simulink model "tx2"  (R2022a)
settings: Solver=FixedStepDiscrete  StartTime=0.0  StopTime=3.1e6  FixedStep=1  RelTol=1e-3
undefined symbols (not defined in the file or in its folder): rom_bf1, rom_bf2, rom_bf3, rom_bf4, rom_bf5, rom_bf6, rom_bf7, rom_bf8, rom_pilot_tt
libraries: hdlsllib x809, whdlutilities x460, whdlmod x104, whdledac x26, simulink x3
(part 10 of 27)

== system tx2/Subsystem11/bit_level/valid_recover ==
  data_in : Inport
  start_in : Inport  Port=2
  end_in : Inport  Port=3
  Constant : Constant  OutDataTypeStr=boolean
  Constant1 : Constant  Value=0  OutDataTypeStr=boolean
  Constant2 : Constant  OutDataTypeStr=boolean
  Constant3 : Constant  Value=0  OutDataTypeStr=boolean
  Constant4 : Constant  OutDataTypeStr=boolean
  Constant5 : Constant  Value=0  OutDataTypeStr=boolean
  Delay{,1..4} (5 alike) : Delay  DelayLength=1  InitialCondition=0
  Logical Operator1 : Logic  Operator=OR  AllPortsSameDT=off  OutDataTypeStr=boolean
  Logical Operator2 : Logic  AllPortsSameDT=off  OutDataTypeStr=boolean
  Switch : Switch  Criteria=u2 ~= 0  SaturateOnIntegerOverflow=off  InputSameDT=off
  Switch1 : Switch  Criteria=u2 ~= 0  SaturateOnIntegerOverflow=off  InputSameDT=off
  Switch2 : Switch  Criteria=u2 ~= 0  SaturateOnIntegerOverflow=off  InputSameDT=off
  data_out : Outport  VectorParamsAs1DForOutWhenUnconnected=off
  start_out : Outport  Port=2  VectorParamsAs1DForOutWhenUnconnected=off
  end_out : Outport  Port=3  VectorParamsAs1DForOutWhenUnconnected=off
  valid_out : Outport  Port=4  VectorParamsAs1DForOutWhenUnconnected=off
  wires:
  Delay4/1 -> data_out/1
  data_in/1 -> Delay4/1
  Delay1/1 -> Delay2/1, end_out/1
  end_in/1 -> Delay1/1
  Constant1/1 -> Switch/3
  Logical Operator2/1 -> Delay3/1, valid_out/1
  Constant3/1 -> Switch1/1
  start_in/1 -> Delay/1
  Constant4/1 -> Switch2/1
  Constant5/1 -> Switch2/3
  Delay3/1 -> Switch2/2
  Switch2/1 -> Logical Operator1/1
  Logical Operator1/1 -> Logical Operator2/1
  Delay2/1 -> Switch1/2
  Delay/1 -> Switch/2, start_out/1
  Switch1/1 -> Logical Operator2/2
  Switch/1 -> Logical Operator1/2
  Constant2/1 -> Switch1/3
  Constant/1 -> Switch/1

== system tx2/Subsystem12/BF/rom_bf1 ==
  address : Inport
  read_en : Inport  Port=2
  HDL ROM : Subsystem
  InputReg : Delay  DelayLength=1  ShowEnablePort=on
      settings: InputPortMap=u0,e6
  data_out : Outport
  wires:
  address/1 -> InputReg/1
  InputReg/1 -> HDL ROM/1(rom_address)
  read_en/1 -> InputReg/2
  HDL ROM/1(data_out) -> data_out/1

== system tx2/Subsystem12/BF/rom_bf2 ==
  address : Inport
  read_en : Inport  Port=2
  HDL ROM : Subsystem
  InputReg : Delay  DelayLength=1  ShowEnablePort=on
      settings: InputPortMap=u0,e6
  data_out : Outport
  wires:
  HDL ROM/1(data_out) -> data_out/1
  read_en/1 -> InputReg/2
  InputReg/1 -> HDL ROM/1(rom_address)
  address/1 -> InputReg/1

== system tx2/Subsystem12/BF/rom_bf3 ==
  address : Inport
  read_en : Inport  Port=2
  HDL ROM : Subsystem
  InputReg : Delay  DelayLength=1  ShowEnablePort=on
      settings: InputPortMap=u0,e6
  data_out : Outport
  wires:
  address/1 -> InputReg/1
  InputReg/1 -> HDL ROM/1(rom_address)
  read_en/1 -> InputReg/2
  HDL ROM/1(data_out) -> data_out/1

== system tx2/Subsystem12/BF/rom_bf4 ==
  address : Inport
  read_en : Inport  Port=2
  HDL ROM : Subsystem
  InputReg : Delay  DelayLength=1  ShowEnablePort=on
      settings: InputPortMap=u0,e6
  data_out : Outport
  wires:
  HDL ROM/1(data_out) -> data_out/1
  read_en/1 -> InputReg/2
  InputReg/1 -> HDL ROM/1(rom_address)
  address/1 -> InputReg/1

== system tx2/Subsystem12/BF/rom_bf5 ==
  address : Inport
  read_en : Inport  Port=2
  HDL ROM : Subsystem
  InputReg : Delay  DelayLength=1  ShowEnablePort=on
      settings: InputPortMap=u0,e6
  data_out : Outport
  wires:
  address/1 -> InputReg/1
  InputReg/1 -> HDL ROM/1(rom_address)
  read_en/1 -> InputReg/2
  HDL ROM/1(data_out) -> data_out/1

== system tx2/Subsystem12/BF/rom_bf6 ==
  address : Inport
  read_en : Inport  Port=2
  HDL ROM : Subsystem
  InputReg : Delay  DelayLength=1  ShowEnablePort=on
      settings: InputPortMap=u0,e6
  data_out : Outport
  wires:
  HDL ROM/1(data_out) -> data_out/1
  read_en/1 -> InputReg/2
  InputReg/1 -> HDL ROM/1(rom_address)
  address/1 -> InputReg/1

== system tx2/Subsystem12/BF/rom_bf7 ==
  address : Inport
  read_en : Inport  Port=2
  HDL ROM : Subsystem
  InputReg : Delay  DelayLength=1  ShowEnablePort=on
      settings: InputPortMap=u0,e6
  data_out : Outport
  wires:
  address/1 -> InputReg/1
  InputReg/1 -> HDL ROM/1(rom_address)
  read_en/1 -> InputReg/2
  HDL ROM/1(data_out) -> data_out/1

== system tx2/Subsystem12/BF/rom_bf8 ==
  address : Inport
  read_en : Inport  Port=2
  HDL ROM : Subsystem
  InputReg : Delay  DelayLength=1  ShowEnablePort=on
      settings: InputPortMap=u0,e6
  data_out : Outport
  wires:
  HDL ROM/1(data_out) -> data_out/1
  read_en/1 -> InputReg/2
  InputReg/1 -> HDL ROM/1(rom_address)
  address/1 -> InputReg/1

== system tx2/Subsystem12/OFDM_process1/OFDM_process1_bf1 ==
  data : Inport
  BF_ctrl : Inport  Port=2
  OFDM_BF1 : Subsystem
  ctrl_gen : Subsystem
  OFDM_process : Outport
  OFDM_ctrl_process : Outport  Port=2
  wires:
  ctrl_gen/1(data_out) -> OFDM_process/1  "OFDM_bf1_process1"
  BF_ctrl/1 -> OFDM_BF1/2(OFDM_ctrl)
  ctrl_gen/2(ctrl_out) -> OFDM_ctrl_process/1  "OFDM_ctrl_bf1_process1"
  data/1 -> OFDM_BF1/1(data)
  OFDM_BF1/2(valid_out) -> ctrl_gen/2(valid_in)
  OFDM_BF1/1(data_out) -> ctrl_gen/1(data_in)

== system tx2/Subsystem12/OFDM_process1/OFDM_process1_bf2 ==
  data : Inport
  BF_ctrl : Inport  Port=2
  OFDM_BF1 : Subsystem
  ctrl_gen : Subsystem
  OFDM_process : Outport
  OFDM_ctrl_process : Outport  Port=2
  wires:
  OFDM_BF1/1(data_out) -> ctrl_gen/1(data_in)
  OFDM_BF1/2(valid_out) -> ctrl_gen/2(valid_in)
  data/1 -> OFDM_BF1/1(data)
  ctrl_gen/2(ctrl_out) -> OFDM_ctrl_process/1  "OFDM_ctrl_bf1_process1"
  BF_ctrl/1 -> OFDM_BF1/2(OFDM_ctrl)
  ctrl_gen/1(data_out) -> OFDM_process/1  "OFDM_bf1_process1"

== system tx2/Subsystem12/OFDM_process1/OFDM_process1_bf3 ==
  data : Inport
  BF_ctrl : Inport  Port=2
  OFDM_BF1 : Subsystem
  ctrl_gen : Subsystem
  OFDM_process : Outport
  OFDM_ctrl_process : Outport  Port=2
  wires:
  ctrl_gen/1(data_out) -> OFDM_process/1  "OFDM_bf1_process1"
  BF_ctrl/1 -> OFDM_BF1/2(OFDM_ctrl)
  ctrl_gen/2(ctrl_out) -> OFDM_ctrl_process/1  "OFDM_ctrl_bf1_process1"
  data/1 -> OFDM_BF1/1(data)
  OFDM_BF1/2(valid_out) -> ctrl_gen/2(valid_in)
  OFDM_BF1/1(data_out) -> ctrl_gen/1(data_in)

== system tx2/Subsystem12/OFDM_process1/OFDM_process1_bf4 ==
  data : Inport
  BF_ctrl : Inport  Port=2
  OFDM_BF1 : Subsystem
  ctrl_gen : Subsystem
  OFDM_process : Outport
  OFDM_ctrl_process : Outport  Port=2
  wires:
  OFDM_BF1/1(data_out) -> ctrl_gen/1(data_in)
  OFDM_BF1/2(valid_out) -> ctrl_gen/2(valid_in)
  data/1 -> OFDM_BF1/1(data)
  ctrl_gen/2(ctrl_out) -> OFDM_ctrl_process/1  "OFDM_ctrl_bf1_process1"
  BF_ctrl/1 -> OFDM_BF1/2(OFDM_ctrl)
  ctrl_gen/1(data_out) -> OFDM_process/1  "OFDM_bf1_process1"

== system tx2/Subsystem12/OFDM_process1/OFDM_process1_bf5 ==
  data : Inport
  BF_ctrl : Inport  Port=2
  OFDM_BF1 : Subsystem
  ctrl_gen : Subsystem
  OFDM_process : Outport
  OFDM_ctrl_process : Outport  Port=2
  wires:
  ctrl_gen/1(data_out) -> OFDM_process/1  "OFDM_bf1_process1"
  BF_ctrl/1 -> OFDM_BF1/2(OFDM_ctrl)
  ctrl_gen/2(ctrl_out) -> OFDM_ctrl_process/1  "OFDM_ctrl_bf1_process1"
  data/1 -> OFDM_BF1/1(data)
  OFDM_BF1/2(valid_out) -> ctrl_gen/2(valid_in)
  OFDM_BF1/1(data_out) -> ctrl_gen/1(data_in)

== system tx2/Subsystem12/OFDM_process1/OFDM_process1_bf6 ==
  data : Inport
  BF_ctrl : Inport  Port=2
  OFDM_BF1 : Subsystem
  ctrl_gen : Subsystem
  OFDM_process : Outport
  OFDM_ctrl_process : Outport  Port=2
  wires:
  OFDM_BF1/1(data_out) -> ctrl_gen/1(data_in)
  OFDM_BF1/2(valid_out) -> ctrl_gen/2(valid_in)
  data/1 -> OFDM_BF1/1(data)
  ctrl_gen/2(ctrl_out) -> OFDM_ctrl_process/1  "OFDM_ctrl_bf1_process1"
  BF_ctrl/1 -> OFDM_BF1/2(OFDM_ctrl)
  ctrl_gen/1(data_out) -> OFDM_process/1  "OFDM_bf1_process1"

== system tx2/Subsystem12/OFDM_process1/OFDM_process1_bf7 ==
  data : Inport
  BF_ctrl : Inport  Port=2
  OFDM_BF1 : Subsystem
  ctrl_gen : Subsystem
  OFDM_process : Outport
  OFDM_ctrl_process : Outport  Port=2
  wires:
  ctrl_gen/1(data_out) -> OFDM_process/1  "OFDM_bf1_process1"
  BF_ctrl/1 -> OFDM_BF1/2(OFDM_ctrl)
  ctrl_gen/2(ctrl_out) -> OFDM_ctrl_process/1  "OFDM_ctrl_bf1_process1"
  data/1 -> OFDM_BF1/1(data)
  OFDM_BF1/2(valid_out) -> ctrl_gen/2(valid_in)
  OFDM_BF1/1(data_out) -> ctrl_gen/1(data_in)

== system tx2/Subsystem12/OFDM_process1/OFDM_process1_bf8 ==
  data : Inport
  BF_ctrl : Inport  Port=2
  OFDM_BF1 : Subsystem
  ctrl_gen : Subsystem
  OFDM_process : Outport
  OFDM_ctrl_process : Outport  Port=2
  wires:
  OFDM_BF1/1(data_out) -> ctrl_gen/1(data_in)
  OFDM_BF1/2(valid_out) -> ctrl_gen/2(valid_in)
  data/1 -> OFDM_BF1/1(data)
  ctrl_gen/2(ctrl_out) -> OFDM_ctrl_process/1  "OFDM_ctrl_bf1_process1"
  BF_ctrl/1 -> OFDM_BF1/2(OFDM_ctrl)
  ctrl_gen/1(data_out) -> OFDM_process/1  "OFDM_bf1_process1"

== system tx2/Subsystem12/bit_level/Subsystem ==
  end_in : Inport  OutDataTypeStr=boolean
  Data Type Conversion : DataTypeConversion  OutDataTypeStr=boolean  SaturateOnIntegerOverflow=off  RndMeth=Floor
  HDL Counter : hdlsllib/Sources/HDL Counter  CountType=Count limited  CountInit=1  CountStep=1  CountMax=192  CountFromType=Initial value  CountFrom=1  CountResetPort=on  CountLoadPort=off  CountEnbPort=off  CountDirPort=off  CountHitOutputPort=on  CountDataType=Unsigned  CountWordLen=8  CountFracLen=0  CountSampTime=1
  HDL Counter1 : hdlsllib/Sources/HDL Counter  CountType=Count limited  CountInit=0  CountStep=1  CountMax=1  CountFromType=Initial value  CountFrom=0  CountResetPort=on  CountLoadPort=off  CountEnbPort=on  CountDirPort=off  CountHitOutputPort=off  CountDataType=Unsigned  CountWordLen=1  CountFracLen=0  CountSampTime=1
  Logical Operator : Logic  AllPortsSameDT=off  OutDataTypeStr=boolean
  end_out : Outport  OutDataTypeStr=boolean
  wires:
  Logical Operator/1 -> end_out/1
  HDL Counter/2 -> HDL Counter1/1, Logical Operator/1
  Data Type Conversion/1 -> Logical Operator/2
  end_in/1 -> HDL Counter1/2, HDL Counter/1
  HDL Counter1/1 -> Data Type Conversion/1

== system tx2/Subsystem12/bit_level/ctrl_gen ==
  data_in : Inport
  select_valid : Inport  Port=2  OutDataTypeStr=boolean
  Constant : Constant  Value=0  OutDataTypeStr=boolean
  Switch : Switch  Criteria=u2 ~= 0  SaturateOnIntegerOverflow=off  InputSameDT=off
  ctrl_gen : Subsystem
  data_out : Outport
  ctrl_out : Outport  Port=2
  wires:
  data_in/1 -> Switch/1
  ctrl_gen/2(ctrl_out) -> ctrl_out/1
  ctrl_gen/1(data_out) -> data_out/1
  select_valid/1 -> Switch/2, ctrl_gen/2(valid_in)
  Constant/1 -> Switch/3
  Switch/1 -> ctrl_gen/1(data_in)

== system tx2/Subsystem12/bit_level/valid_recover ==
  data_in : Inport
  start_in : Inport  Port=2
  end_in : Inport  Port=3
  Constant : Constant  OutDataTypeStr=boolean
  Constant1 : Constant  Value=0  OutDataTypeStr=boolean
  Constant2 : Constant  OutDataTypeStr=boolean
  Constant3 : Constant  Value=0  OutDataTypeStr=boolean
  Constant4 : Constant  OutDataTypeStr=boolean
  Constant5 : Constant  Value=0  OutDataTypeStr=boolean
  Delay{,1..4} (5 alike) : Delay  DelayLength=1  InitialCondition=0
  Logical Operator1 : Logic  Operator=OR  AllPortsSameDT=off  OutDataTypeStr=boolean
  Logical Operator2 : Logic  AllPortsSameDT=off  OutDataTypeStr=boolean
  Switch : Switch  Criteria=u2 ~= 0  SaturateOnIntegerOverflow=off  InputSameDT=off
  Switch1 : Switch  Criteria=u2 ~= 0  SaturateOnIntegerOverflow=off  InputSameDT=off
  Switch2 : Switch  Criteria=u2 ~= 0  SaturateOnIntegerOverflow=off  InputSameDT=off
  data_out : Outport  VectorParamsAs1DForOutWhenUnconnected=off
  start_out : Outport  Port=2  VectorParamsAs1DForOutWhenUnconnected=off
  end_out : Outport  Port=3  VectorParamsAs1DForOutWhenUnconnected=off
  valid_out : Outport  Port=4  VectorParamsAs1DForOutWhenUnconnected=off
  wires:
  Constant/1 -> Switch/1
  Constant2/1 -> Switch1/3
  Switch/1 -> Logical Operator1/2
  Switch1/1 -> Logical Operator2/2
  Delay/1 -> start_out/1, Switch/2
  Delay2/1 -> Switch1/2
  Logical Operator1/1 -> Logical Operator2/1
  Switch2/1 -> Logical Operator1/1
  Delay3/1 -> Switch2/2
  Constant5/1 -> Switch2/3
  Constant4/1 -> Switch2/1
  start_in/1 -> Delay/1
  Constant3/1 -> Switch1/1
  Logical Operator2/1 -> valid_out/1, Delay3/1
  Constant1/1 -> Switch/3
  end_in/1 -> Delay1/1
  Delay1/1 -> end_out/1, Delay2/1
  data_in/1 -> Delay4/1
  Delay4/1 -> data_out/1

== system tx2/Subsystem13/BF/rom_bf1 ==
  address : Inport
  read_en : Inport  Port=2
  HDL ROM : Subsystem
  InputReg : Delay  DelayLength=1  ShowEnablePort=on
      settings: InputPortMap=u0,e6
  data_out : Outport
  wires:
  address/1 -> InputReg/1
  InputReg/1 -> HDL ROM/1(rom_address)
  read_en/1 -> InputReg/2
  HDL ROM/1(data_out) -> data_out/1

== system tx2/Subsystem13/BF/rom_bf2 ==
  address : Inport
  read_en : Inport  Port=2
  HDL ROM : Subsystem
  InputReg : Delay  DelayLength=1  ShowEnablePort=on
      settings: InputPortMap=u0,e6
  data_out : Outport
  wires:
  HDL ROM/1(data_out) -> data_out/1
  read_en/1 -> InputReg/2
  InputReg/1 -> HDL ROM/1(rom_address)
  address/1 -> InputReg/1

== system tx2/Subsystem13/BF/rom_bf3 ==
  address : Inport
  read_en : Inport  Port=2
  HDL ROM : Subsystem
  InputReg : Delay  DelayLength=1  ShowEnablePort=on
      settings: InputPortMap=u0,e6
  data_out : Outport
  wires:
  address/1 -> InputReg/1
  InputReg/1 -> HDL ROM/1(rom_address)
  read_en/1 -> InputReg/2
  HDL ROM/1(data_out) -> data_out/1

== system tx2/Subsystem13/BF/rom_bf4 ==
  address : Inport
  read_en : Inport  Port=2
  HDL ROM : Subsystem
  InputReg : Delay  DelayLength=1  ShowEnablePort=on
      settings: InputPortMap=u0,e6
  data_out : Outport
  wires:
  HDL ROM/1(data_out) -> data_out/1
  read_en/1 -> InputReg/2
  InputReg/1 -> HDL ROM/1(rom_address)
  address/1 -> InputReg/1

== system tx2/Subsystem13/BF/rom_bf5 ==
  address : Inport
  read_en : Inport  Port=2
  HDL ROM : Subsystem
  InputReg : Delay  DelayLength=1  ShowEnablePort=on
      settings: InputPortMap=u0,e6
  data_out : Outport
  wires:
  address/1 -> InputReg/1
  InputReg/1 -> HDL ROM/1(rom_address)
  read_en/1 -> InputReg/2
  HDL ROM/1(data_out) -> data_out/1

== system tx2/Subsystem13/BF/rom_bf6 ==
  address : Inport
  read_en : Inport  Port=2
  HDL ROM : Subsystem
  InputReg : Delay  DelayLength=1  ShowEnablePort=on
      settings: InputPortMap=u0,e6
  data_out : Outport
  wires:
  HDL ROM/1(data_out) -> data_out/1
  read_en/1 -> InputReg/2
  InputReg/1 -> HDL ROM/1(rom_address)
  address/1 -> InputReg/1

== system tx2/Subsystem13/BF/rom_bf7 ==
  address : Inport
  read_en : Inport  Port=2
  HDL ROM : Subsystem
  InputReg : Delay  DelayLength=1  ShowEnablePort=on
      settings: InputPortMap=u0,e6
  data_out : Outport
  wires:
  address/1 -> InputReg/1
  InputReg/1 -> HDL ROM/1(rom_address)
  read_en/1 -> InputReg/2
  HDL ROM/1(data_out) -> data_out/1

== system tx2/Subsystem13/BF/rom_bf8 ==
  address : Inport
  read_en : Inport  Port=2
  HDL ROM : Subsystem
  InputReg : Delay  DelayLength=1  ShowEnablePort=on
      settings: InputPortMap=u0,e6
  data_out : Outport
  wires:
  HDL ROM/1(data_out) -> data_out/1
  read_en/1 -> InputReg/2
  InputReg/1 -> HDL ROM/1(rom_address)
  address/1 -> InputReg/1

== system tx2/Subsystem13/OFDM_process1/OFDM_process1_bf1 ==
  data : Inport
  BF_ctrl : Inport  Port=2
  OFDM_BF1 : Subsystem
  ctrl_gen : Subsystem
  OFDM_process : Outport
  OFDM_ctrl_process : Outport  Port=2
  wires:
  OFDM_BF1/1(data_out) -> ctrl_gen/1(data_in)
  OFDM_BF1/2(valid_out) -> ctrl_gen/2(valid_in)
  data/1 -> OFDM_BF1/1(data)
  ctrl_gen/2(ctrl_out) -> OFDM_ctrl_process/1  "OFDM_ctrl_bf1_process1"
  BF_ctrl/1 -> OFDM_BF1/2(OFDM_ctrl)
  ctrl_gen/1(data_out) -> OFDM_process/1  "OFDM_bf1_process1"

== system tx2/Subsystem13/OFDM_process1/OFDM_process1_bf2 ==
  data : Inport
  BF_ctrl : Inport  Port=2
  OFDM_BF1 : Subsystem
  ctrl_gen : Subsystem
  OFDM_process : Outport
  OFDM_ctrl_process : Outport  Port=2
  wires:
  ctrl_gen/1(data_out) -> OFDM_process/1  "OFDM_bf1_process1"
  BF_ctrl/1 -> OFDM_BF1/2(OFDM_ctrl)
  ctrl_gen/2(ctrl_out) -> OFDM_ctrl_process/1  "OFDM_ctrl_bf1_process1"
  data/1 -> OFDM_BF1/1(data)
  OFDM_BF1/2(valid_out) -> ctrl_gen/2(valid_in)
  OFDM_BF1/1(data_out) -> ctrl_gen/1(data_in)

== system tx2/Subsystem13/OFDM_process1/OFDM_process1_bf3 ==
  data : Inport
  BF_ctrl : Inport  Port=2
  OFDM_BF1 : Subsystem
  ctrl_gen : Subsystem
  OFDM_process : Outport
  OFDM_ctrl_process : Outport  Port=2
  wires:
  OFDM_BF1/1(data_out) -> ctrl_gen/1(data_in)
  OFDM_BF1/2(valid_out) -> ctrl_gen/2(valid_in)
  data/1 -> OFDM_BF1/1(data)
  ctrl_gen/2(ctrl_out) -> OFDM_ctrl_process/1  "OFDM_ctrl_bf1_process1"
  BF_ctrl/1 -> OFDM_BF1/2(OFDM_ctrl)
  ctrl_gen/1(data_out) -> OFDM_process/1  "OFDM_bf1_process1"

== system tx2/Subsystem13/OFDM_process1/OFDM_process1_bf4 ==
  data : Inport
  BF_ctrl : Inport  Port=2
  OFDM_BF1 : Subsystem
  ctrl_gen : Subsystem
  OFDM_process : Outport
  OFDM_ctrl_process : Outport  Port=2
  wires:
  ctrl_gen/1(data_out) -> OFDM_process/1  "OFDM_bf1_process1"
  BF_ctrl/1 -> OFDM_BF1/2(OFDM_ctrl)
  ctrl_gen/2(ctrl_out) -> OFDM_ctrl_process/1  "OFDM_ctrl_bf1_process1"
  data/1 -> OFDM_BF1/1(data)
  OFDM_BF1/2(valid_out) -> ctrl_gen/2(valid_in)
  OFDM_BF1/1(data_out) -> ctrl_gen/1(data_in)

== system tx2/Subsystem13/OFDM_process1/OFDM_process1_bf5 ==
  data : Inport
  BF_ctrl : Inport  Port=2
  OFDM_BF1 : Subsystem
  ctrl_gen : Subsystem
  OFDM_process : Outport
  OFDM_ctrl_process : Outport  Port=2
  wires:
  OFDM_BF1/1(data_out) -> ctrl_gen/1(data_in)
  OFDM_BF1/2(valid_out) -> ctrl_gen/2(valid_in)
  data/1 -> OFDM_BF1/1(data)
  ctrl_gen/2(ctrl_out) -> OFDM_ctrl_process/1  "OFDM_ctrl_bf1_process1"
  BF_ctrl/1 -> OFDM_BF1/2(OFDM_ctrl)
  ctrl_gen/1(data_out) -> OFDM_process/1  "OFDM_bf1_process1"

== system tx2/Subsystem13/OFDM_process1/OFDM_process1_bf6 ==
  data : Inport
  BF_ctrl : Inport  Port=2
  OFDM_BF1 : Subsystem
  ctrl_gen : Subsystem
  OFDM_process : Outport
  OFDM_ctrl_process : Outport  Port=2
  wires:
  ctrl_gen/1(data_out) -> OFDM_process/1  "OFDM_bf1_process1"
  BF_ctrl/1 -> OFDM_BF1/2(OFDM_ctrl)
  ctrl_gen/2(ctrl_out) -> OFDM_ctrl_process/1  "OFDM_ctrl_bf1_process1"
  data/1 -> OFDM_BF1/1(data)
  OFDM_BF1/2(valid_out) -> ctrl_gen/2(valid_in)
  OFDM_BF1/1(data_out) -> ctrl_gen/1(data_in)

== system tx2/Subsystem13/OFDM_process1/OFDM_process1_bf7 ==
  data : Inport
  BF_ctrl : Inport  Port=2
  OFDM_BF1 : Subsystem
  ctrl_gen : Subsystem
  OFDM_process : Outport
  OFDM_ctrl_process : Outport  Port=2
  wires:
  OFDM_BF1/1(data_out) -> ctrl_gen/1(data_in)
  OFDM_BF1/2(valid_out) -> ctrl_gen/2(valid_in)
  data/1 -> OFDM_BF1/1(data)
  ctrl_gen/2(ctrl_out) -> OFDM_ctrl_process/1  "OFDM_ctrl_bf1_process1"
  BF_ctrl/1 -> OFDM_BF1/2(OFDM_ctrl)
  ctrl_gen/1(data_out) -> OFDM_process/1  "OFDM_bf1_process1"

== system tx2/Subsystem13/OFDM_process1/OFDM_process1_bf8 ==
  data : Inport
  BF_ctrl : Inport  Port=2
  OFDM_BF1 : Subsystem
  ctrl_gen : Subsystem
  OFDM_process : Outport
  OFDM_ctrl_process : Outport  Port=2
  wires:
  ctrl_gen/1(data_out) -> OFDM_process/1  "OFDM_bf1_process1"
  BF_ctrl/1 -> OFDM_BF1/2(OFDM_ctrl)
  ctrl_gen/2(ctrl_out) -> OFDM_ctrl_process/1  "OFDM_ctrl_bf1_process1"
  data/1 -> OFDM_BF1/1(data)
  OFDM_BF1/2(valid_out) -> ctrl_gen/2(valid_in)
  OFDM_BF1/1(data_out) -> ctrl_gen/1(data_in)

== system tx2/Subsystem13/bit_level/Subsystem ==
  end_in : Inport  OutDataTypeStr=boolean
  Data Type Conversion : DataTypeConversion  OutDataTypeStr=boolean  SaturateOnIntegerOverflow=off  RndMeth=Floor
  HDL Counter : hdlsllib/Sources/HDL Counter  CountType=Count limited  CountInit=1  CountStep=1  CountMax=192  CountFromType=Initial value  CountFrom=1  CountResetPort=on  CountLoadPort=off  CountEnbPort=off  CountDirPort=off  CountHitOutputPort=on  CountDataType=Unsigned  CountWordLen=8  CountFracLen=0  CountSampTime=1
  HDL Counter1 : hdlsllib/Sources/HDL Counter  CountType=Count limited  CountInit=0  CountStep=1  CountMax=1  CountFromType=Initial value  CountFrom=0  CountResetPort=on  CountLoadPort=off  CountEnbPort=on  CountDirPort=off  CountHitOutputPort=off  CountDataType=Unsigned  CountWordLen=1  CountFracLen=0  CountSampTime=1
  Logical Operator : Logic  AllPortsSameDT=off  OutDataTypeStr=boolean
  end_out : Outport  OutDataTypeStr=boolean
  wires:
  HDL Counter1/1 -> Data Type Conversion/1
  end_in/1 -> HDL Counter/1, HDL Counter1/2
  Data Type Conversion/1 -> Logical Operator/2
  HDL Counter/2 -> Logical Operator/1, HDL Counter1/1
  Logical Operator/1 -> end_out/1

== system tx2/Subsystem13/bit_level/ctrl_gen ==
  data_in : Inport
  select_valid : Inport  Port=2  OutDataTypeStr=boolean
  Constant : Constant  Value=0  OutDataTypeStr=boolean
  Switch : Switch  Criteria=u2 ~= 0  SaturateOnIntegerOverflow=off  InputSameDT=off
  ctrl_gen : Subsystem
  data_out : Outport
  ctrl_out : Outport  Port=2
  wires:
  Switch/1 -> ctrl_gen/1(data_in)
  Constant/1 -> Switch/3
  select_valid/1 -> ctrl_gen/2(valid_in), Switch/2
  ctrl_gen/1(data_out) -> data_out/1
  ctrl_gen/2(ctrl_out) -> ctrl_out/1
  data_in/1 -> Switch/1

== system tx2/Subsystem13/bit_level/valid_recover ==
  data_in : Inport
  start_in : Inport  Port=2
  end_in : Inport  Port=3
  Constant : Constant  OutDataTypeStr=boolean
  Constant1 : Constant  Value=0  OutDataTypeStr=boolean
  Constant2 : Constant  OutDataTypeStr=boolean
  Constant3 : Constant  Value=0  OutDataTypeStr=boolean
  Constant4 : Constant  OutDataTypeStr=boolean
  Constant5 : Constant  Value=0  OutDataTypeStr=boolean
  Delay{,1..4} (5 alike) : Delay  DelayLength=1  InitialCondition=0
  Logical Operator1 : Logic  Operator=OR  AllPortsSameDT=off  OutDataTypeStr=boolean
  Logical Operator2 : Logic  AllPortsSameDT=off  OutDataTypeStr=boolean
  Switch : Switch  Criteria=u2 ~= 0  SaturateOnIntegerOverflow=off  InputSameDT=off
  Switch1 : Switch  Criteria=u2 ~= 0  SaturateOnIntegerOverflow=off  InputSameDT=off
  Switch2 : Switch  Criteria=u2 ~= 0  SaturateOnIntegerOverflow=off  InputSameDT=off
  data_out : Outport  VectorParamsAs1DForOutWhenUnconnected=off
  start_out : Outport  Port=2  VectorParamsAs1DForOutWhenUnconnected=off
  end_out : Outport  Port=3  VectorParamsAs1DForOutWhenUnconnected=off
  valid_out : Outport  Port=4  VectorParamsAs1DForOutWhenUnconnected=off
  wires:
  Delay4/1 -> data_out/1
  data_in/1 -> Delay4/1
  Delay1/1 -> Delay2/1, end_out/1
  end_in/1 -> Delay1/1
  Constant1/1 -> Switch/3
  Logical Operator2/1 -> Delay3/1, valid_out/1
  Constant3/1 -> Switch1/1
  start_in/1 -> Delay/1
  Constant4/1 -> Switch2/1
  Constant5/1 -> Switch2/3
  Delay3/1 -> Switch2/2
  Switch2/1 -> Logical Operator1/1
  Logical Operator1/1 -> Logical Operator2/1
  Delay2/1 -> Switch1/2
  Delay/1 -> Switch/2, start_out/1
  Switch1/1 -> Logical Operator2/2
  Switch/1 -> Logical Operator1/2
  Constant2/1 -> Switch1/3
  Constant/1 -> Switch/1

== system tx2/Subsystem2/BF/rom_bf1 ==
  address : Inport
  read_en : Inport  Port=2
  HDL ROM : Subsystem
  InputReg : Delay  DelayLength=1  ShowEnablePort=on
      settings: InputPortMap=u0,e6
  data_out : Outport
  wires:
  address/1 -> InputReg/1
  InputReg/1 -> HDL ROM/1(rom_address)
  read_en/1 -> InputReg/2
  HDL ROM/1(data_out) -> data_out/1

== system tx2/Subsystem2/BF/rom_bf2 ==
  address : Inport
  read_en : Inport  Port=2
  HDL ROM : Subsystem
  InputReg : Delay  DelayLength=1  ShowEnablePort=on
      settings: InputPortMap=u0,e6
  data_out : Outport
  wires:
  HDL ROM/1(data_out) -> data_out/1
  read_en/1 -> InputReg/2
  InputReg/1 -> HDL ROM/1(rom_address)
  address/1 -> InputReg/1

== system tx2/Subsystem2/BF/rom_bf3 ==
  address : Inport
  read_en : Inport  Port=2
  HDL ROM : Subsystem
  InputReg : Delay  DelayLength=1  ShowEnablePort=on
      settings: InputPortMap=u0,e6
  data_out : Outport
  wires:
  address/1 -> InputReg/1
  InputReg/1 -> HDL ROM/1(rom_address)
  read_en/1 -> InputReg/2
  HDL ROM/1(data_out) -> data_out/1

== system tx2/Subsystem2/BF/rom_bf4 ==
  address : Inport
  read_en : Inport  Port=2
  HDL ROM : Subsystem
  InputReg : Delay  DelayLength=1  ShowEnablePort=on
      settings: InputPortMap=u0,e6
  data_out : Outport
  wires:
  HDL ROM/1(data_out) -> data_out/1
  read_en/1 -> InputReg/2
  InputReg/1 -> HDL ROM/1(rom_address)
  address/1 -> InputReg/1

== system tx2/Subsystem2/BF/rom_bf5 ==
  address : Inport
  read_en : Inport  Port=2
  HDL ROM : Subsystem
  InputReg : Delay  DelayLength=1  ShowEnablePort=on
      settings: InputPortMap=u0,e6
  data_out : Outport
  wires:
  address/1 -> InputReg/1
  InputReg/1 -> HDL ROM/1(rom_address)
  read_en/1 -> InputReg/2
  HDL ROM/1(data_out) -> data_out/1

== system tx2/Subsystem2/BF/rom_bf6 ==
  address : Inport
  read_en : Inport  Port=2
  HDL ROM : Subsystem
  InputReg : Delay  DelayLength=1  ShowEnablePort=on
      settings: InputPortMap=u0,e6
  data_out : Outport
  wires:
  HDL ROM/1(data_out) -> data_out/1
  read_en/1 -> InputReg/2
  InputReg/1 -> HDL ROM/1(rom_address)
  address/1 -> InputReg/1

== system tx2/Subsystem2/BF/rom_bf7 ==
  address : Inport
  read_en : Inport  Port=2
  HDL ROM : Subsystem
  InputReg : Delay  DelayLength=1  ShowEnablePort=on
      settings: InputPortMap=u0,e6
  data_out : Outport
  wires:
  address/1 -> InputReg/1
  InputReg/1 -> HDL ROM/1(rom_address)
  read_en/1 -> InputReg/2
  HDL ROM/1(data_out) -> data_out/1

== system tx2/Subsystem2/BF/rom_bf8 ==
  address : Inport
  read_en : Inport  Port=2
  HDL ROM : Subsystem
  InputReg : Delay  DelayLength=1  ShowEnablePort=on
      settings: InputPortMap=u0,e6
  data_out : Outport
  wires:
  HDL ROM/1(data_out) -> data_out/1
  read_en/1 -> InputReg/2
  InputReg/1 -> HDL ROM/1(rom_address)
  address/1 -> InputReg/1

== system tx2/Subsystem2/OFDM_process1/OFDM_process1_bf1 ==
  data : Inport
  BF_ctrl : Inport  Port=2
  OFDM_BF1 : Subsystem
  ctrl_gen : Subsystem
  OFDM_process : Outport
  OFDM_ctrl_process : Outport  Port=2
  wires:
  ctrl_gen/1(data_out) -> OFDM_process/1  "OFDM_bf1_process1"
  BF_ctrl/1 -> OFDM_BF1/2(OFDM_ctrl)
  ctrl_gen/2(ctrl_out) -> OFDM_ctrl_process/1  "OFDM_ctrl_bf1_process1"
  data/1 -> OFDM_BF1/1(data)
  OFDM_BF1/2(valid_out) -> ctrl_gen/2(valid_in)
  OFDM_BF1/1(data_out) -> ctrl_gen/1(data_in)

== system tx2/Subsystem2/OFDM_process1/OFDM_process1_bf2 ==
  data : Inport
  BF_ctrl : Inport  Port=2
  OFDM_BF1 : Subsystem
  ctrl_gen : Subsystem
  OFDM_process : Outport
  OFDM_ctrl_process : Outport  Port=2
  wires:
  OFDM_BF1/1(data_out) -> ctrl_gen/1(data_in)
  OFDM_BF1/2(valid_out) -> ctrl_gen/2(valid_in)
  data/1 -> OFDM_BF1/1(data)
  ctrl_gen/2(ctrl_out) -> OFDM_ctrl_process/1  "OFDM_ctrl_bf1_process1"
  BF_ctrl/1 -> OFDM_BF1/2(OFDM_ctrl)
  ctrl_gen/1(data_out) -> OFDM_process/1  "OFDM_bf1_process1"

== system tx2/Subsystem2/OFDM_process1/OFDM_process1_bf3 ==
  data : Inport
  BF_ctrl : Inport  Port=2
  OFDM_BF1 : Subsystem
  ctrl_gen : Subsystem
  OFDM_process : Outport
  OFDM_ctrl_process : Outport  Port=2
  wires:
  ctrl_gen/1(data_out) -> OFDM_process/1  "OFDM_bf1_process1"
  BF_ctrl/1 -> OFDM_BF1/2(OFDM_ctrl)
  ctrl_gen/2(ctrl_out) -> OFDM_ctrl_process/1  "OFDM_ctrl_bf1_process1"
  data/1 -> OFDM_BF1/1(data)
  OFDM_BF1/2(valid_out) -> ctrl_gen/2(valid_in)
  OFDM_BF1/1(data_out) -> ctrl_gen/1(data_in)

== system tx2/Subsystem2/OFDM_process1/OFDM_process1_bf4 ==
  data : Inport
  BF_ctrl : Inport  Port=2
  OFDM_BF1 : Subsystem
  ctrl_gen : Subsystem
  OFDM_process : Outport
  OFDM_ctrl_process : Outport  Port=2
  wires:
  OFDM_BF1/1(data_out) -> ctrl_gen/1(data_in)
  OFDM_BF1/2(valid_out) -> ctrl_gen/2(valid_in)
  data/1 -> OFDM_BF1/1(data)
  ctrl_gen/2(ctrl_out) -> OFDM_ctrl_process/1  "OFDM_ctrl_bf1_process1"
  BF_ctrl/1 -> OFDM_BF1/2(OFDM_ctrl)
  ctrl_gen/1(data_out) -> OFDM_process/1  "OFDM_bf1_process1"

== system tx2/Subsystem2/OFDM_process1/OFDM_process1_bf5 ==
  data : Inport
  BF_ctrl : Inport  Port=2
  OFDM_BF1 : Subsystem
  ctrl_gen : Subsystem
  OFDM_process : Outport
  OFDM_ctrl_process : Outport  Port=2
  wires:
  ctrl_gen/1(data_out) -> OFDM_process/1  "OFDM_bf1_process1"
  BF_ctrl/1 -> OFDM_BF1/2(OFDM_ctrl)
  ctrl_gen/2(ctrl_out) -> OFDM_ctrl_process/1  "OFDM_ctrl_bf1_process1"
  data/1 -> OFDM_BF1/1(data)
  OFDM_BF1/2(valid_out) -> ctrl_gen/2(valid_in)
  OFDM_BF1/1(data_out) -> ctrl_gen/1(data_in)

== system tx2/Subsystem2/OFDM_process1/OFDM_process1_bf6 ==
  data : Inport
  BF_ctrl : Inport  Port=2
  OFDM_BF1 : Subsystem
  ctrl_gen : Subsystem
  OFDM_process : Outport
  OFDM_ctrl_process : Outport  Port=2
  wires:
  OFDM_BF1/1(data_out) -> ctrl_gen/1(data_in)
  OFDM_BF1/2(valid_out) -> ctrl_gen/2(valid_in)
  data/1 -> OFDM_BF1/1(data)
  ctrl_gen/2(ctrl_out) -> OFDM_ctrl_process/1  "OFDM_ctrl_bf1_process1"
  BF_ctrl/1 -> OFDM_BF1/2(OFDM_ctrl)
  ctrl_gen/1(data_out) -> OFDM_process/1  "OFDM_bf1_process1"

== system tx2/Subsystem2/OFDM_process1/OFDM_process1_bf7 ==
  data : Inport
  BF_ctrl : Inport  Port=2
  OFDM_BF1 : Subsystem
  ctrl_gen : Subsystem
  OFDM_process : Outport
  OFDM_ctrl_process : Outport  Port=2
  wires:
  ctrl_gen/1(data_out) -> OFDM_process/1  "OFDM_bf1_process1"
  BF_ctrl/1 -> OFDM_BF1/2(OFDM_ctrl)
  ctrl_gen/2(ctrl_out) -> OFDM_ctrl_process/1  "OFDM_ctrl_bf1_process1"
  data/1 -> OFDM_BF1/1(data)
  OFDM_BF1/2(valid_out) -> ctrl_gen/2(valid_in)
  OFDM_BF1/1(data_out) -> ctrl_gen/1(data_in)

== system tx2/Subsystem2/OFDM_process1/OFDM_process1_bf8 ==
  data : Inport
  BF_ctrl : Inport  Port=2
  OFDM_BF1 : Subsystem
  ctrl_gen : Subsystem
  OFDM_process : Outport
  OFDM_ctrl_process : Outport  Port=2
  wires:
  OFDM_BF1/1(data_out) -> ctrl_gen/1(data_in)
  OFDM_BF1/2(valid_out) -> ctrl_gen/2(valid_in)
  data/1 -> OFDM_BF1/1(data)
  ctrl_gen/2(ctrl_out) -> OFDM_ctrl_process/1  "OFDM_ctrl_bf1_process1"
  BF_ctrl/1 -> OFDM_BF1/2(OFDM_ctrl)
  ctrl_gen/1(data_out) -> OFDM_process/1  "OFDM_bf1_process1"

== system tx2/Subsystem2/bit_level/Subsystem ==
  end_in : Inport  OutDataTypeStr=boolean
  Data Type Conversion : DataTypeConversion  OutDataTypeStr=boolean  SaturateOnIntegerOverflow=off  RndMeth=Floor
  HDL Counter : hdlsllib/Sources/HDL Counter  CountType=Count limited  CountInit=1  CountStep=1  CountMax=192  CountFromType=Initial value  CountFrom=1  CountResetPort=on  CountLoadPort=off  CountEnbPort=off  CountDirPort=off  CountHitOutputPort=on  CountDataType=Unsigned  CountWordLen=8  CountFracLen=0  CountSampTime=1
  HDL Counter1 : hdlsllib/Sources/HDL Counter  CountType=Count limited  CountInit=0  CountStep=1  CountMax=1  CountFromType=Initial value  CountFrom=0  CountResetPort=on  CountLoadPort=off  CountEnbPort=on  CountDirPort=off  CountHitOutputPort=off  CountDataType=Unsigned  CountWordLen=1  CountFracLen=0  CountSampTime=1
  Logical Operator : Logic  AllPortsSameDT=off  OutDataTypeStr=boolean
  end_out : Outport  OutDataTypeStr=boolean
  wires:
  Logical Operator/1 -> end_out/1
  HDL Counter/2 -> HDL Counter1/1, Logical Operator/1
  Data Type Conversion/1 -> Logical Operator/2
  end_in/1 -> HDL Counter1/2, HDL Counter/1
  HDL Counter1/1 -> Data Type Conversion/1

== system tx2/Subsystem2/bit_level/ctrl_gen ==
  data_in : Inport
  select_valid : Inport  Port=2  OutDataTypeStr=boolean
  Constant : Constant  Value=0  OutDataTypeStr=boolean
  Switch : Switch  Criteria=u2 ~= 0  SaturateOnIntegerOverflow=off  InputSameDT=off
  ctrl_gen : Subsystem
  data_out : Outport
  ctrl_out : Outport  Port=2
  wires:
  data_in/1 -> Switch/1
  ctrl_gen/2(ctrl_out) -> ctrl_out/1
  ctrl_gen/1(data_out) -> data_out/1
  select_valid/1 -> Switch/2, ctrl_gen/2(valid_in)
  Constant/1 -> Switch/3
  Switch/1 -> ctrl_gen/1(data_in)

== system tx2/Subsystem2/bit_level/valid_recover ==
  data_in : Inport
  start_in : Inport  Port=2
  end_in : Inport  Port=3
  Constant : Constant  OutDataTypeStr=boolean
  Constant1 : Constant  Value=0  OutDataTypeStr=boolean
  Constant2 : Constant  OutDataTypeStr=boolean
  Constant3 : Constant  Value=0  OutDataTypeStr=boolean
  Constant4 : Constant  OutDataTypeStr=boolean
  Constant5 : Constant  Value=0  OutDataTypeStr=boolean
  Delay{,1..4} (5 alike) : Delay  DelayLength=1  InitialCondition=0
  Logical Operator1 : Logic  Operator=OR  AllPortsSameDT=off  OutDataTypeStr=boolean
  Logical Operator2 : Logic  AllPortsSameDT=off  OutDataTypeStr=boolean
  Switch : Switch  Criteria=u2 ~= 0  SaturateOnIntegerOverflow=off  InputSameDT=off
  Switch1 : Switch  Criteria=u2 ~= 0  SaturateOnIntegerOverflow=off  InputSameDT=off
  Switch2 : Switch  Criteria=u2 ~= 0  SaturateOnIntegerOverflow=off  InputSameDT=off
  data_out : Outport  VectorParamsAs1DForOutWhenUnconnected=off
  start_out : Outport  Port=2  VectorParamsAs1DForOutWhenUnconnected=off
  end_out : Outport  Port=3  VectorParamsAs1DForOutWhenUnconnected=off
  valid_out : Outport  Port=4  VectorParamsAs1DForOutWhenUnconnected=off
  wires:
  Constant/1 -> Switch/1
  Constant2/1 -> Switch1/3
  Switch/1 -> Logical Operator1/2
  Switch1/1 -> Logical Operator2/2
  Delay/1 -> start_out/1, Switch/2
  Delay2/1 -> Switch1/2
  Logical Operator1/1 -> Logical Operator2/1
  Switch2/1 -> Logical Operator1/1
  Delay3/1 -> Switch2/2
  Constant5/1 -> Switch2/3
  Constant4/1 -> Switch2/1
  start_in/1 -> Delay/1
  Constant3/1 -> Switch1/1
  Logical Operator2/1 -> valid_out/1, Delay3/1
  Constant1/1 -> Switch/3
  end_in/1 -> Delay1/1
  Delay1/1 -> end_out/1, Delay2/1
  data_in/1 -> Delay4/1
  Delay4/1 -> data_out/1

== system tx2/Subsystem3/BF/rom_bf1 ==
  address : Inport
  read_en : Inport  Port=2
  HDL ROM : Subsystem
  InputReg : Delay  DelayLength=1  ShowEnablePort=on
      settings: InputPortMap=u0,e6
  data_out : Outport
  wires:
  address/1 -> InputReg/1
  InputReg/1 -> HDL ROM/1(rom_address)
  read_en/1 -> InputReg/2
  HDL ROM/1(data_out) -> data_out/1

== system tx2/Subsystem3/BF/rom_bf2 ==
  address : Inport
  read_en : Inport  Port=2
  HDL ROM : Subsystem
  InputReg : Delay  DelayLength=1  ShowEnablePort=on
      settings: InputPortMap=u0,e6
  data_out : Outport
  wires:
  HDL ROM/1(data_out) -> data_out/1
  read_en/1 -> InputReg/2
  InputReg/1 -> HDL ROM/1(rom_address)
  address/1 -> InputReg/1

== system tx2/Subsystem3/BF/rom_bf3 ==
  address : Inport
  read_en : Inport  Port=2
  HDL ROM : Subsystem
  InputReg : Delay  DelayLength=1  ShowEnablePort=on
      settings: InputPortMap=u0,e6
  data_out : Outport
  wires:
  address/1 -> InputReg/1
  InputReg/1 -> HDL ROM/1(rom_address)
  read_en/1 -> InputReg/2
  HDL ROM/1(data_out) -> data_out/1

== system tx2/Subsystem3/BF/rom_bf4 ==
  address : Inport
  read_en : Inport  Port=2
  HDL ROM : Subsystem
  InputReg : Delay  DelayLength=1  ShowEnablePort=on
      settings: InputPortMap=u0,e6
  data_out : Outport
  wires:
  HDL ROM/1(data_out) -> data_out/1
  read_en/1 -> InputReg/2
  InputReg/1 -> HDL ROM/1(rom_address)
  address/1 -> InputReg/1

== system tx2/Subsystem3/BF/rom_bf5 ==
  address : Inport
  read_en : Inport  Port=2
  HDL ROM : Subsystem
  InputReg : Delay  DelayLength=1  ShowEnablePort=on
      settings: InputPortMap=u0,e6
  data_out : Outport
  wires:
  address/1 -> InputReg/1
  InputReg/1 -> HDL ROM/1(rom_address)
  read_en/1 -> InputReg/2
  HDL ROM/1(data_out) -> data_out/1

== system tx2/Subsystem3/BF/rom_bf6 ==
  address : Inport
  read_en : Inport  Port=2
  HDL ROM : Subsystem
  InputReg : Delay  DelayLength=1  ShowEnablePort=on
      settings: InputPortMap=u0,e6
  data_out : Outport
  wires:
  HDL ROM/1(data_out) -> data_out/1
  read_en/1 -> InputReg/2
  InputReg/1 -> HDL ROM/1(rom_address)
  address/1 -> InputReg/1

== system tx2/Subsystem3/BF/rom_bf7 ==
  address : Inport
  read_en : Inport  Port=2
  HDL ROM : Subsystem
  InputReg : Delay  DelayLength=1  ShowEnablePort=on
      settings: InputPortMap=u0,e6
  data_out : Outport
  wires:
  address/1 -> InputReg/1
  InputReg/1 -> HDL ROM/1(rom_address)
  read_en/1 -> InputReg/2
  HDL ROM/1(data_out) -> data_out/1

== system tx2/Subsystem3/BF/rom_bf8 ==
  address : Inport
  read_en : Inport  Port=2
  HDL ROM : Subsystem
  InputReg : Delay  DelayLength=1  ShowEnablePort=on
      settings: InputPortMap=u0,e6
  data_out : Outport
  wires:
  HDL ROM/1(data_out) -> data_out/1
  read_en/1 -> InputReg/2
  InputReg/1 -> HDL ROM/1(rom_address)
  address/1 -> InputReg/1

== system tx2/Subsystem3/OFDM_process1/OFDM_process1_bf1 ==
  data : Inport
  BF_ctrl : Inport  Port=2
  OFDM_BF1 : Subsystem
  ctrl_gen : Subsystem
  OFDM_process : Outport
  OFDM_ctrl_process : Outport  Port=2
  wires:
  OFDM_BF1/1(data_out) -> ctrl_gen/1(data_in)
  OFDM_BF1/2(valid_out) -> ctrl_gen/2(valid_in)
  data/1 -> OFDM_BF1/1(data)
  ctrl_gen/2(ctrl_out) -> OFDM_ctrl_process/1  "OFDM_ctrl_bf1_process1"
  BF_ctrl/1 -> OFDM_BF1/2(OFDM_ctrl)
  ctrl_gen/1(data_out) -> OFDM_process/1  "OFDM_bf1_process1"

== system tx2/Subsystem3/OFDM_process1/OFDM_process1_bf2 ==
  data : Inport
  BF_ctrl : Inport  Port=2
  OFDM_BF1 : Subsystem
  ctrl_gen : Subsystem
  OFDM_process : Outport
  OFDM_ctrl_process : Outport  Port=2
  wires:
  ctrl_gen/1(data_out) -> OFDM_process/1  "OFDM_bf1_process1"
  BF_ctrl/1 -> OFDM_BF1/2(OFDM_ctrl)
  ctrl_gen/2(ctrl_out) -> OFDM_ctrl_process/1  "OFDM_ctrl_bf1_process1"
  data/1 -> OFDM_BF1/1(data)
  OFDM_BF1/2(valid_out) -> ctrl_gen/2(valid_in)
  OFDM_BF1/1(data_out) -> ctrl_gen/1(data_in)

== system tx2/Subsystem3/OFDM_process1/OFDM_process1_bf3 ==
  data : Inport
  BF_ctrl : Inport  Port=2
  OFDM_BF1 : Subsystem
  ctrl_gen : Subsystem
  OFDM_process : Outport
  OFDM_ctrl_process : Outport  Port=2
  wires:
  OFDM_BF1/1(data_out) -> ctrl_gen/1(data_in)
  OFDM_BF1/2(valid_out) -> ctrl_gen/2(valid_in)
  data/1 -> OFDM_BF1/1(data)
  ctrl_gen/2(ctrl_out) -> OFDM_ctrl_process/1  "OFDM_ctrl_bf1_process1"
  BF_ctrl/1 -> OFDM_BF1/2(OFDM_ctrl)
  ctrl_gen/1(data_out) -> OFDM_process/1  "OFDM_bf1_process1"

== system tx2/Subsystem3/OFDM_process1/OFDM_process1_bf4 ==
  data : Inport
  BF_ctrl : Inport  Port=2
  OFDM_BF1 : Subsystem
  ctrl_gen : Subsystem
  OFDM_process : Outport
  OFDM_ctrl_process : Outport  Port=2
  wires:
  ctrl_gen/1(data_out) -> OFDM_process/1  "OFDM_bf1_process1"
  BF_ctrl/1 -> OFDM_BF1/2(OFDM_ctrl)
  ctrl_gen/2(ctrl_out) -> OFDM_ctrl_process/1  "OFDM_ctrl_bf1_process1"
  data/1 -> OFDM_BF1/1(data)
  OFDM_BF1/2(valid_out) -> ctrl_gen/2(valid_in)
  OFDM_BF1/1(data_out) -> ctrl_gen/1(data_in)

== system tx2/Subsystem3/OFDM_process1/OFDM_process1_bf5 ==
  data : Inport
  BF_ctrl : Inport  Port=2
  OFDM_BF1 : Subsystem
  ctrl_gen : Subsystem
  OFDM_process : Outport
  OFDM_ctrl_process : Outport  Port=2
  wires:
  OFDM_BF1/1(data_out) -> ctrl_gen/1(data_in)
  OFDM_BF1/2(valid_out) -> ctrl_gen/2(valid_in)
  data/1 -> OFDM_BF1/1(data)
  ctrl_gen/2(ctrl_out) -> OFDM_ctrl_process/1  "OFDM_ctrl_bf1_process1"
  BF_ctrl/1 -> OFDM_BF1/2(OFDM_ctrl)
  ctrl_gen/1(data_out) -> OFDM_process/1  "OFDM_bf1_process1"

== system tx2/Subsystem3/OFDM_process1/OFDM_process1_bf6 ==
  data : Inport
  BF_ctrl : Inport  Port=2
  OFDM_BF1 : Subsystem
  ctrl_gen : Subsystem
  OFDM_process : Outport
  OFDM_ctrl_process : Outport  Port=2
  wires:
  ctrl_gen/1(data_out) -> OFDM_process/1  "OFDM_bf1_process1"
  BF_ctrl/1 -> OFDM_BF1/2(OFDM_ctrl)
  ctrl_gen/2(ctrl_out) -> OFDM_ctrl_process/1  "OFDM_ctrl_bf1_process1"
  data/1 -> OFDM_BF1/1(data)
  OFDM_BF1/2(valid_out) -> ctrl_gen/2(valid_in)
  OFDM_BF1/1(data_out) -> ctrl_gen/1(data_in)

== system tx2/Subsystem3/OFDM_process1/OFDM_process1_bf7 ==
  data : Inport
  BF_ctrl : Inport  Port=2
  OFDM_BF1 : Subsystem
  ctrl_gen : Subsystem
  OFDM_process : Outport
  OFDM_ctrl_process : Outport  Port=2
  wires:
  OFDM_BF1/1(data_out) -> ctrl_gen/1(data_in)
  OFDM_BF1/2(valid_out) -> ctrl_gen/2(valid_in)
  data/1 -> OFDM_BF1/1(data)
  ctrl_gen/2(ctrl_out) -> OFDM_ctrl_process/1  "OFDM_ctrl_bf1_process1"
  BF_ctrl/1 -> OFDM_BF1/2(OFDM_ctrl)
  ctrl_gen/1(data_out) -> OFDM_process/1  "OFDM_bf1_process1"

== system tx2/Subsystem3/OFDM_process1/OFDM_process1_bf8 ==
  data : Inport
  BF_ctrl : Inport  Port=2
  OFDM_BF1 : Subsystem
  ctrl_gen : Subsystem
  OFDM_process : Outport
  OFDM_ctrl_process : Outport  Port=2
  wires:
  ctrl_gen/1(data_out) -> OFDM_process/1  "OFDM_bf1_process1"
  BF_ctrl/1 -> OFDM_BF1/2(OFDM_ctrl)
  ctrl_gen/2(ctrl_out) -> OFDM_ctrl_process/1  "OFDM_ctrl_bf1_process1"
  data/1 -> OFDM_BF1/1(data)
  OFDM_BF1/2(valid_out) -> ctrl_gen/2(valid_in)
  OFDM_BF1/1(data_out) -> ctrl_gen/1(data_in)

== system tx2/Subsystem3/bit_level/Subsystem ==
  end_in : Inport  OutDataTypeStr=boolean
  Data Type Conversion : DataTypeConversion  OutDataTypeStr=boolean  SaturateOnIntegerOverflow=off  RndMeth=Floor
  HDL Counter : hdlsllib/Sources/HDL Counter  CountType=Count limited  CountInit=1  CountStep=1  CountMax=192  CountFromType=Initial value  CountFrom=1  CountResetPort=on  CountLoadPort=off  CountEnbPort=off  CountDirPort=off  CountHitOutputPort=on  CountDataType=Unsigned  CountWordLen=8  CountFracLen=0  CountSampTime=1
  HDL Counter1 : hdlsllib/Sources/HDL Counter  CountType=Count limited  CountInit=0  CountStep=1  CountMax=1  CountFromType=Initial value  CountFrom=0  CountResetPort=on  CountLoadPort=off  CountEnbPort=on  CountDirPort=off  CountHitOutputPort=off  CountDataType=Unsigned  CountWordLen=1  CountFracLen=0  CountSampTime=1
  Logical Operator : Logic  AllPortsSameDT=off  OutDataTypeStr=boolean
  end_out : Outport  OutDataTypeStr=boolean
  wires:
  HDL Counter1/1 -> Data Type Conversion/1
  end_in/1 -> HDL Counter/1, HDL Counter1/2
  Data Type Conversion/1 -> Logical Operator/2
  HDL Counter/2 -> Logical Operator/1, HDL Counter1/1
  Logical Operator/1 -> end_out/1

== system tx2/Subsystem3/bit_level/ctrl_gen ==
  data_in : Inport
  select_valid : Inport  Port=2  OutDataTypeStr=boolean
  Constant : Constant  Value=0  OutDataTypeStr=boolean
  Switch : Switch  Criteria=u2 ~= 0  SaturateOnIntegerOverflow=off  InputSameDT=off
  ctrl_gen : Subsystem
  data_out : Outport
  ctrl_out : Outport  Port=2
  wires:
  Switch/1 -> ctrl_gen/1(data_in)
  Constant/1 -> Switch/3
  select_valid/1 -> ctrl_gen/2(valid_in), Switch/2
  ctrl_gen/1(data_out) -> data_out/1
  ctrl_gen/2(ctrl_out) -> ctrl_out/1
  data_in/1 -> Switch/1

== system tx2/Subsystem3/bit_level/valid_recover ==
  data_in : Inport
  start_in : Inport  Port=2
  end_in : Inport  Port=3
  Constant : Constant  OutDataTypeStr=boolean
  Constant1 : Constant  Value=0  OutDataTypeStr=boolean
  Constant2 : Constant  OutDataTypeStr=boolean
  Constant3 : Constant  Value=0  OutDataTypeStr=boolean
  Constant4 : Constant  OutDataTypeStr=boolean
  Constant5 : Constant  Value=0  OutDataTypeStr=boolean
  Delay{,1..4} (5 alike) : Delay  DelayLength=1  InitialCondition=0
  Logical Operator1 : Logic  Operator=OR  AllPortsSameDT=off  OutDataTypeStr=boolean
  Logical Operator2 : Logic  AllPortsSameDT=off  OutDataTypeStr=boolean
  Switch : Switch  Criteria=u2 ~= 0  SaturateOnIntegerOverflow=off  InputSameDT=off
  Switch1 : Switch  Criteria=u2 ~= 0  SaturateOnIntegerOverflow=off  InputSameDT=off
  Switch2 : Switch  Criteria=u2 ~= 0  SaturateOnIntegerOverflow=off  InputSameDT=off
  data_out : Outport  VectorParamsAs1DForOutWhenUnconnected=off
  start_out : Outport  Port=2  VectorParamsAs1DForOutWhenUnconnected=off
  end_out : Outport  Port=3  VectorParamsAs1DForOutWhenUnconnected=off
  valid_out : Outport  Port=4  VectorParamsAs1DForOutWhenUnconnected=off
  wires:
  Delay4/1 -> data_out/1
  data_in/1 -> Delay4/1
  Delay1/1 -> Delay2/1, end_out/1
  end_in/1 -> Delay1/1
  Constant1/1 -> Switch/3
  Logical Operator2/1 -> Delay3/1, valid_out/1
  Constant3/1 -> Switch1/1
  start_in/1 -> Delay/1
  Constant4/1 -> Switch2/1
  Constant5/1 -> Switch2/3
  Delay3/1 -> Switch2/2
  Switch2/1 -> Logical Operator1/1
  Logical Operator1/1 -> Logical Operator2/1
  Delay2/1 -> Switch1/2
  Delay/1 -> Switch/2, start_out/1
  Switch1/1 -> Logical Operator2/2
  Switch/1 -> Logical Operator1/2
  Constant2/1 -> Switch1/3
  Constant/1 -> Switch/1

== system tx2/Subsystem4/BF/rom_bf1 ==
  address : Inport
  read_en : Inport  Port=2
  HDL ROM : Subsystem
  InputReg : Delay  DelayLength=1  ShowEnablePort=on
      settings: InputPortMap=u0,e6
  data_out : Outport
  wires:
  address/1 -> InputReg/1
  InputReg/1 -> HDL ROM/1(rom_address)
  read_en/1 -> InputReg/2
  HDL ROM/1(data_out) -> data_out/1

== system tx2/Subsystem4/BF/rom_bf2 ==
  address : Inport
  read_en : Inport  Port=2
  HDL ROM : Subsystem
  InputReg : Delay  DelayLength=1  ShowEnablePort=on
      settings: InputPortMap=u0,e6
  data_out : Outport
  wires:
  HDL ROM/1(data_out) -> data_out/1
  read_en/1 -> InputReg/2
  InputReg/1 -> HDL ROM/1(rom_address)
  address/1 -> InputReg/1

== system tx2/Subsystem4/BF/rom_bf3 ==
  address : Inport
  read_en : Inport  Port=2
  HDL ROM : Subsystem
  InputReg : Delay  DelayLength=1  ShowEnablePort=on
      settings: InputPortMap=u0,e6
  data_out : Outport
  wires:
  address/1 -> InputReg/1
  InputReg/1 -> HDL ROM/1(rom_address)
  read_en/1 -> InputReg/2
  HDL ROM/1(data_out) -> data_out/1

== system tx2/Subsystem4/BF/rom_bf4 ==
  address : Inport
  read_en : Inport  Port=2
  HDL ROM : Subsystem
  InputReg : Delay  DelayLength=1  ShowEnablePort=on
      settings: InputPortMap=u0,e6
  data_out : Outport
  wires:
  HDL ROM/1(data_out) -> data_out/1
  read_en/1 -> InputReg/2
  InputReg/1 -> HDL ROM/1(rom_address)
  address/1 -> InputReg/1

== system tx2/Subsystem4/BF/rom_bf5 ==
  address : Inport
  read_en : Inport  Port=2
  HDL ROM : Subsystem
  InputReg : Delay  DelayLength=1  ShowEnablePort=on
      settings: InputPortMap=u0,e6
  data_out : Outport
  wires:
  address/1 -> InputReg/1
  InputReg/1 -> HDL ROM/1(rom_address)
  read_en/1 -> InputReg/2
  HDL ROM/1(data_out) -> data_out/1

== system tx2/Subsystem4/BF/rom_bf6 ==
  address : Inport
  read_en : Inport  Port=2
  HDL ROM : Subsystem
  InputReg : Delay  DelayLength=1  ShowEnablePort=on
      settings: InputPortMap=u0,e6
  data_out : Outport
  wires:
  HDL ROM/1(data_out) -> data_out/1
  read_en/1 -> InputReg/2
  InputReg/1 -> HDL ROM/1(rom_address)
  address/1 -> InputReg/1

== system tx2/Subsystem4/BF/rom_bf7 ==
  address : Inport
  read_en : Inport  Port=2
  HDL ROM : Subsystem
  InputReg : Delay  DelayLength=1  ShowEnablePort=on
      settings: InputPortMap=u0,e6
  data_out : Outport
  wires:
  address/1 -> InputReg/1
  InputReg/1 -> HDL ROM/1(rom_address)
  read_en/1 -> InputReg/2
  HDL ROM/1(data_out) -> data_out/1

== system tx2/Subsystem4/BF/rom_bf8 ==
  address : Inport
  read_en : Inport  Port=2
  HDL ROM : Subsystem
  InputReg : Delay  DelayLength=1  ShowEnablePort=on
      settings: InputPortMap=u0,e6
  data_out : Outport
  wires:
  HDL ROM/1(data_out) -> data_out/1
  read_en/1 -> InputReg/2
  InputReg/1 -> HDL ROM/1(rom_address)
  address/1 -> InputReg/1

== system tx2/Subsystem4/OFDM_process1/OFDM_process1_bf1 ==
  data : Inport
  BF_ctrl : Inport  Port=2
  OFDM_BF1 : Subsystem
  ctrl_gen : Subsystem
  OFDM_process : Outport
  OFDM_ctrl_process : Outport  Port=2
  wires:
  ctrl_gen/1(data_out) -> OFDM_process/1  "OFDM_bf1_process1"
  BF_ctrl/1 -> OFDM_BF1/2(OFDM_ctrl)
  ctrl_gen/2(ctrl_out) -> OFDM_ctrl_process/1  "OFDM_ctrl_bf1_process1"
  data/1 -> OFDM_BF1/1(data)
  OFDM_BF1/2(valid_out) -> ctrl_gen/2(valid_in)
  OFDM_BF1/1(data_out) -> ctrl_gen/1(data_in)

== system tx2/Subsystem4/OFDM_process1/OFDM_process1_bf2 ==
  data : Inport
  BF_ctrl : Inport  Port=2
  OFDM_BF1 : Subsystem
  ctrl_gen : Subsystem
  OFDM_process : Outport
  OFDM_ctrl_process : Outport  Port=2
  wires:
  OFDM_BF1/1(data_out) -> ctrl_gen/1(data_in)
  OFDM_BF1/2(valid_out) -> ctrl_gen/2(valid_in)
  data/1 -> OFDM_BF1/1(data)
  ctrl_gen/2(ctrl_out) -> OFDM_ctrl_process/1  "OFDM_ctrl_bf1_process1"
  BF_ctrl/1 -> OFDM_BF1/2(OFDM_ctrl)
  ctrl_gen/1(data_out) -> OFDM_process/1  "OFDM_bf1_process1"

== system tx2/Subsystem4/OFDM_process1/OFDM_process1_bf3 ==
  data : Inport
  BF_ctrl : Inport  Port=2
  OFDM_BF1 : Subsystem
  ctrl_gen : Subsystem
  OFDM_process : Outport
  OFDM_ctrl_process : Outport  Port=2
  wires:
  ctrl_gen/1(data_out) -> OFDM_process/1  "OFDM_bf1_process1"
  BF_ctrl/1 -> OFDM_BF1/2(OFDM_ctrl)
  ctrl_gen/2(ctrl_out) -> OFDM_ctrl_process/1  "OFDM_ctrl_bf1_process1"
  data/1 -> OFDM_BF1/1(data)
  OFDM_BF1/2(valid_out) -> ctrl_gen/2(valid_in)
  OFDM_BF1/1(data_out) -> ctrl_gen/1(data_in)

== system tx2/Subsystem4/OFDM_process1/OFDM_process1_bf4 ==
  data : Inport
  BF_ctrl : Inport  Port=2
  OFDM_BF1 : Subsystem
  ctrl_gen : Subsystem
  OFDM_process : Outport
  OFDM_ctrl_process : Outport  Port=2
  wires:
  OFDM_BF1/1(data_out) -> ctrl_gen/1(data_in)
  OFDM_BF1/2(valid_out) -> ctrl_gen/2(valid_in)
  data/1 -> OFDM_BF1/1(data)
  ctrl_gen/2(ctrl_out) -> OFDM_ctrl_process/1  "OFDM_ctrl_bf1_process1"
  BF_ctrl/1 -> OFDM_BF1/2(OFDM_ctrl)
  ctrl_gen/1(data_out) -> OFDM_process/1  "OFDM_bf1_process1"

== system tx2/Subsystem4/OFDM_process1/OFDM_process1_bf5 ==
  data : Inport
  BF_ctrl : Inport  Port=2
  OFDM_BF1 : Subsystem
  ctrl_gen : Subsystem
  OFDM_process : Outport
  OFDM_ctrl_process : Outport  Port=2
  wires:
  ctrl_gen/1(data_out) -> OFDM_process/1  "OFDM_bf1_process1"
  BF_ctrl/1 -> OFDM_BF1/2(OFDM_ctrl)
  ctrl_gen/2(ctrl_out) -> OFDM_ctrl_process/1  "OFDM_ctrl_bf1_process1"
  data/1 -> OFDM_BF1/1(data)
  OFDM_BF1/2(valid_out) -> ctrl_gen/2(valid_in)
  OFDM_BF1/1(data_out) -> ctrl_gen/1(data_in)

== system tx2/Subsystem4/OFDM_process1/OFDM_process1_bf6 ==
  data : Inport
  BF_ctrl : Inport  Port=2
  OFDM_BF1 : Subsystem
  ctrl_gen : Subsystem
  OFDM_process : Outport
  OFDM_ctrl_process : Outport  Port=2
  wires:
  OFDM_BF1/1(data_out) -> ctrl_gen/1(data_in)
  OFDM_BF1/2(valid_out) -> ctrl_gen/2(valid_in)
  data/1 -> OFDM_BF1/1(data)
  ctrl_gen/2(ctrl_out) -> OFDM_ctrl_process/1  "OFDM_ctrl_bf1_process1"
  BF_ctrl/1 -> OFDM_BF1/2(OFDM_ctrl)
  ctrl_gen/1(data_out) -> OFDM_process/1  "OFDM_bf1_process1"
